simulink model "UNM_TrafficSignalFollower"  (R2025b)
settings: Solver=FixedStepAuto  StartTime=0  StopTime=1000  FixedStep=Ts  RelTol=1e-3
PostLoadFcn:
  | UNM_Setup()
InitFcn:
  | rrHDMap = rrSim.get("Map");
values from neighbouring files (symbols this model uses):
  Ts = 0.1    [SurrogateTrafficEnv.m]    (also in SurrogateTrafficEnvACC.m; UNMTrafficSignalFollower_Block.m; UNM_AccelToSpeed.m; UNM_TrafficSignalVisualization.m = 0.05)
undefined symbols (not defined in the file or in its folder): ActorRuntime, Defined, Ego, Lane, m, n, User
libraries: roadrunnerscenario x11, rllib x1
CloseFcn:
  | clear egoActorID signalID Ts
settings Model: Creator=user  LastModifiedBy=user
settings DataIOCC: InspectSignalLogs=on
settings DebuggingCC: AlgebraicLoopMsg=none

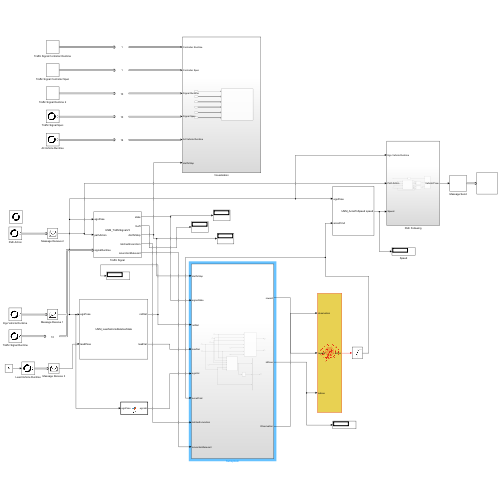
[thumbnail: Simulink's stored preview of the top-level diagram]
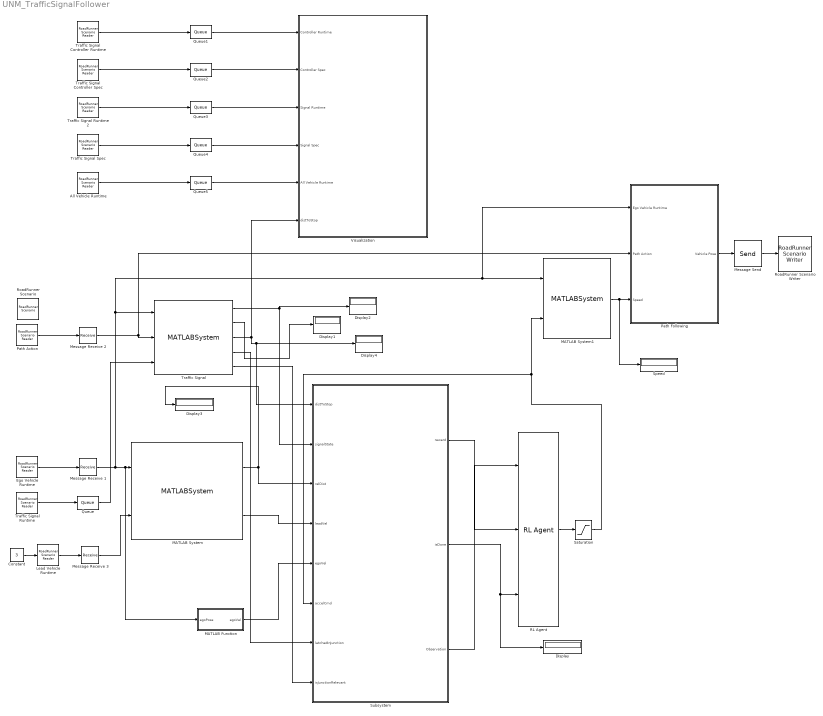
== system UNM_TrafficSignalFollower ==
  All Vehicle Runtime : roadrunnerscenario/RoadRunner Scenario Reader  TopicCategory=Actor  ActorCategory=Vehicle  ActionType=Path Following  EventType=User-Defined  TopicType=Actor Specifications  VehicleType=Vehicle Pose  TrafficSignalType=Traffic Signal Runtime  TrafficSignalControllerType=Traffic Signal Controller Specifications  UserDefinedAction=Action1  UserDefinedEvent=Event1  Filter=None  AdditionalRelationship=None  SensorTopic=Target Poses  LaneBoundaryOutputTopic=Ego-Lane  SensorID=1  SampleTime=Ts
  Constant : Constant  Value=3  OutDataTypeStr=uint64
  Display{,1..4} (5 alike) : Display
  Ego Vehicle Runtime : roadrunnerscenario/RoadRunner Scenario Reader  TopicCategory=Actor  ActorCategory=Vehicle  ActionType=Path Following  EventType=User-Defined  TopicType=Actor Specifications  VehicleType=Vehicle Pose  TrafficSignalType=Traffic Signal Specifications  TrafficSignalControllerType=Traffic Signal Controller Specifications  UserDefinedAction=Action1  UserDefinedEvent=Event1  Filter=Self  AdditionalRelationship=None  SensorTopic=Target Poses  LaneBoundaryOutputTopic=Ego-Lane  SensorID=1  SampleTime=Ts
  Lead Vehicle Runtime : roadrunnerscenario/RoadRunner Scenario Reader  TopicCategory=Actor  ActorCategory=Vehicle  ActionType=Path Following  EventType=User-Defined  TopicType=Actor Specifications  VehicleType=Vehicle Pose  TrafficSignalType=Traffic Signal Specifications  TrafficSignalControllerType=Traffic Signal Controller Specifications  UserDefinedAction=Action1  UserDefinedEvent=Event1  Filter=Actor ID (provided by input)  AdditionalRelationship=None  SensorTopic=Target Poses  LaneBoundaryOutputTopic=Ego-Lane  SensorID=1  SampleTime=Ts
  MATLAB Function : MATLAB Function  TreatAsAtomicUnit=on
  MATLAB System : MATLABSystem  System=UNM_LeadVehicleRelativeState
      mask Type: UNM_LeadVehicleRelativeState
  MATLAB System1 : MATLABSystem  System=UNM_AccelToSpeed  Ts=0.1  MaxSpeed=15
      mask Type: UNM_AccelToSpeed
  "Message Receive 1 " : Receive  InputPortMessageModes=m  UseInternalQueue=off  QueueOverwriting=on  QueueLength=1  QueueType=LIFO
  Message Receive 2 : Receive  InputPortMessageModes=m
  Message Receive 3 : Receive  InputPortMessageModes=m  UseInternalQueue=off  QueueOverwriting=on  QueueLength=1  QueueType=LIFO
  Message Send : Send  OutputPortMessageModes=m
  Path Action : roadrunnerscenario/RoadRunner Scenario Reader  TopicCategory=Action  ActorCategory=All Types  ActionType=Path Following  EventType=User-Defined  TopicType=Actor Specifications  VehicleType=Vehicle Specifications  TrafficSignalType=Traffic Signal Specifications  TrafficSignalControllerType=Traffic Signal Controller Specifications  UserDefinedAction=Action1  UserDefinedEvent=Event1  Filter=Self  AdditionalRelationship=None  SensorTopic=Target Poses  LaneBoundaryOutputTopic=Ego-Lane  SensorID=1  SampleTime=Ts
  Path Following : Subsystem
  Queue : Queue  InputPortMessageModes=m  OutputPortMessageModes=m  OverwriteOldest=on  Capacity=10
  Queue1 : Queue  InputPortMessageModes=m  OutputPortMessageModes=m  OverwriteOldest=on  Capacity=1
  Queue2 : Queue  InputPortMessageModes=m  OutputPortMessageModes=m  OverwriteOldest=on  Capacity=1
  Queue3 : Queue  InputPortMessageModes=m  OutputPortMessageModes=m  OverwriteOldest=on  Capacity=10
  Queue4 : Queue  InputPortMessageModes=m  OutputPortMessageModes=m  OverwriteOldest=on  Capacity=10
  Queue5 : Queue  InputPortMessageModes=m  OutputPortMessageModes=m  OverwriteOldest=on  Capacity=16
  RL Agent : rllib/RL Agent  Agent=agent  ExternalActionAsInput=off  ProvideLastAction=off  ProvideCumRwd=off  TreatAsDirectFeedthrough=on  UseStrictObservationDataTypes=off
  RoadRunner Scenario : roadrunnerscenario/RoadRunner Scenario  UserDefinedActions={}  UserDefinedEvents={}  PathPoints=500
  RoadRunner Scenario Writer : roadrunnerscenario/RoadRunner Scenario Writer  TopicCategory=Actor  ActorCategory=Vehicle  EventType=Action Complete  UserDefinedEvent=Event1  VehicleType=Vehicle Pose  TopicType=Actor Pose
  Saturation : Saturate  UpperLimit=2  LowerLimit=-3
  Speed : Display
  Subsystem : Subsystem
  Traffic Signal : MATLABSystem  InputPortMessageModes=n,n,m  System=UNM_TrafficSignalV3  SignalID=signalID  EgoID=egoActorID  RRHDMap=rrHDMap  MaxStopDistance=100  MaxPhaseDuration=60
      mask Type: UNM_TrafficSignalV3
  Traffic Signal Controller Runtime : roadrunnerscenario/RoadRunner Scenario Reader  TopicCategory=Actor  ActorCategory=Traffic Signal Controller  ActionType=Path Following  EventType=User-Defined  TopicType=Actor Specifications  VehicleType=Vehicle Pose  TrafficSignalType=Traffic Signal Runtime  TrafficSignalControllerType=Traffic Signal Controller Runtime  UserDefinedAction=Action1  UserDefinedEvent=Event1  Filter=None  AdditionalRelationship=None  SensorTopic=Target Poses  LaneBoundaryOutputTopic=Ego-Lane  SensorID=1  SampleTime=Ts
  Traffic Signal Controller Spec : roadrunnerscenario/RoadRunner Scenario Reader  TopicCategory=Actor  ActorCategory=Traffic Signal Controller  ActionType=Path Following  EventType=User-Defined  TopicType=Actor Specifications  VehicleType=Vehicle Pose  TrafficSignalType=Traffic Signal Runtime  TrafficSignalControllerType=Traffic Signal Controller Specifications  UserDefinedAction=Action1  UserDefinedEvent=Event1  Filter=None  AdditionalRelationship=None  SensorTopic=Target Poses  LaneBoundaryOutputTopic=Ego-Lane  SensorID=1  SampleTime=10
  Traffic Signal Runtime : roadrunnerscenario/RoadRunner Scenario Reader  TopicCategory=Actor  ActorCategory=Traffic Signal  ActionType=Path Following  EventType=User-Defined  TopicType=Actor Specifications  VehicleType=Vehicle Pose  TrafficSignalType=Traffic Signal Runtime  TrafficSignalControllerType=Traffic Signal Controller Specifications  UserDefinedAction=Action1  UserDefinedEvent=Event1  Filter=None  AdditionalRelationship=None  SensorTopic=Target Poses  LaneBoundaryOutputTopic=Ego-Lane  SensorID=1  SampleTime=Ts
  Traffic Signal Runtime 2 : roadrunnerscenario/RoadRunner Scenario Reader  TopicCategory=Actor  ActorCategory=Traffic Signal  ActionType=Path Following  EventType=User-Defined  TopicType=Actor Specifications  VehicleType=Vehicle Pose  TrafficSignalType=Traffic Signal Runtime  TrafficSignalControllerType=Traffic Signal Controller Specifications  UserDefinedAction=Action1  UserDefinedEvent=Event1  Filter=None  AdditionalRelationship=None  SensorTopic=Target Poses  LaneBoundaryOutputTopic=Ego-Lane  SensorID=1  SampleTime=Ts
  Traffic Signal Spec : roadrunnerscenario/RoadRunner Scenario Reader  TopicCategory=Actor  ActorCategory=Traffic Signal  ActionType=Path Following  EventType=User-Defined  TopicType=Actor Specifications  VehicleType=Vehicle Pose  TrafficSignalType=Traffic Signal Specifications  TrafficSignalControllerType=Traffic Signal Controller Specifications  UserDefinedAction=Action1  UserDefinedEvent=Event1  Filter=None  AdditionalRelationship=None  SensorTopic=Target Poses  LaneBoundaryOutputTopic=Ego-Lane  SensorID=1  SampleTime=10
  Visualization : Subsystem
  wires:
  Traffic Signal Spec/1 -> Queue4/1
  Message Receive 2/1 -> Path Following/2(Path Action), Traffic Signal/2
  Traffic Signal Runtime 2/1 -> Queue3/1
  Traffic Signal Runtime/1 -> Queue/1
  Message Send/1 -> RoadRunner Scenario Writer/1
  Path Action/1 -> Message Receive 2/1
  Ego Vehicle Runtime/1 -> "Message Receive 1 "/1
  Traffic Signal Controller Spec/1 -> Queue2/1
  "Message Receive 1 "/1 -> Path Following/1(Ego Vehicle Runtime), MATLAB System1/1, Traffic Signal/1, MATLAB Function/1(egoPose), MATLAB System/1
  Traffic Signal Controller Runtime/1 -> Queue1/1
  All Vehicle Runtime/1 -> Queue5/1
  Queue/1 -> Traffic Signal/3
  Queue1/1 -> Visualization/1(Controller Runtime)
  Queue2/1 -> Visualization/2(Controller Spec)
  Queue3/1 -> Visualization/3(Signal Runtime)
  RL Agent/1 -> Saturation/1
  Queue4/1 -> Visualization/4(Signal Spec)
  Traffic Signal/1 -> Subsystem/2(signalState), Display2/1
  Queue5/1 -> Visualization/5(All Vehicle Runtime)
  Saturation/1 -> MATLAB System1/2, Subsystem/6(accelCmd)
  Traffic Signal/2 -> Display1/1
  Traffic Signal/3 -> Subsystem/1(distToStop), Display4/1, Visualization/6(distToStop)
  MATLAB System/1 -> Display3/1, Subsystem/3(relDist)
  Subsystem/1(reward) -> RL Agent/2
  Subsystem/2(isDone) -> RL Agent/3, Display/1
  Subsystem/3(Observation) -> RL Agent/1
  MATLAB System1/1 -> Speed/1, Path Following/3(Speed)
  Path Following/1(Vehicle Pose) -> Message Send/1
  Constant/1 -> Lead Vehicle Runtime/1
  Lead Vehicle Runtime/1 -> Message Receive 3/1
  Message Receive 3/1 -> MATLAB System/2
  MATLAB System/2 -> Subsystem/4(leadVel)
  MATLAB Function/1(egoVel) -> Subsystem/5(egoVel)
  Traffic Signal/4 -> Subsystem/7(latchedInJunction)
  Traffic Signal/5 -> Subsystem/8(isJunctionRelevant)

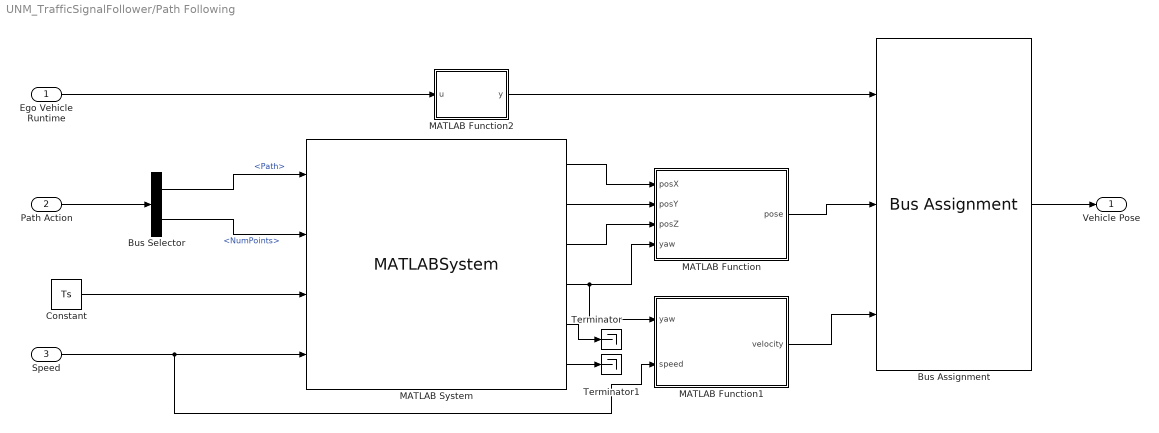
== system UNM_TrafficSignalFollower/Path Following ==
  Ego Vehicle Runtime : Inport
  Path Action : Inport  Port=2
  Speed : Inport  Port=3
  Bus Assignment : BusAssignment  AssignedSignals=ActorRuntime.Pose,ActorRuntime.Velocity
  Bus Selector : BusSelector  OutputSignals=PathTarget.Path,PathTarget.NumPoints
  Constant : Constant  Value=Ts
  MATLAB Function : MATLAB Function  TreatAsAtomicUnit=on
  MATLAB Function1 : MATLAB Function  TreatAsAtomicUnit=on
  MATLAB Function2 : MATLAB Function  TreatAsAtomicUnit=on
  MATLAB System : MATLABSystem  System=UNMPathEvaluator_Block  SimulateUsing=Code generation
      mask Type: UNMPathEvaluator_Block
  Terminator : Terminator
  Terminator1 : Terminator
  Vehicle Pose : Outport
  wires:
  Bus Assignment/1 -> Vehicle Pose/1
  Path Action/1 -> Bus Selector/1
  Constant/1 -> MATLAB System/3
  Speed/1 -> MATLAB Function1/2(speed), MATLAB System/4
  MATLAB Function1/1(velocity) -> Bus Assignment/3
  MATLAB System/1 -> MATLAB Function/1(posX)
  MATLAB Function/1(pose) -> Bus Assignment/2
  MATLAB System/2 -> MATLAB Function/2(posY)
  MATLAB System/3 -> MATLAB Function/3(posZ)
  MATLAB System/4 -> MATLAB Function/4(yaw), MATLAB Function1/1(yaw)
  MATLAB System/5 -> Terminator/1
  MATLAB System/6 -> Terminator1/1
  Bus Selector/1 -> MATLAB System/1  "<Path>"
  Bus Selector/2 -> MATLAB System/2  "<NumPoints>"
  Ego Vehicle Runtime/1 -> MATLAB Function2/1(u)
  MATLAB Function2/1(y) -> Bus Assignment/1

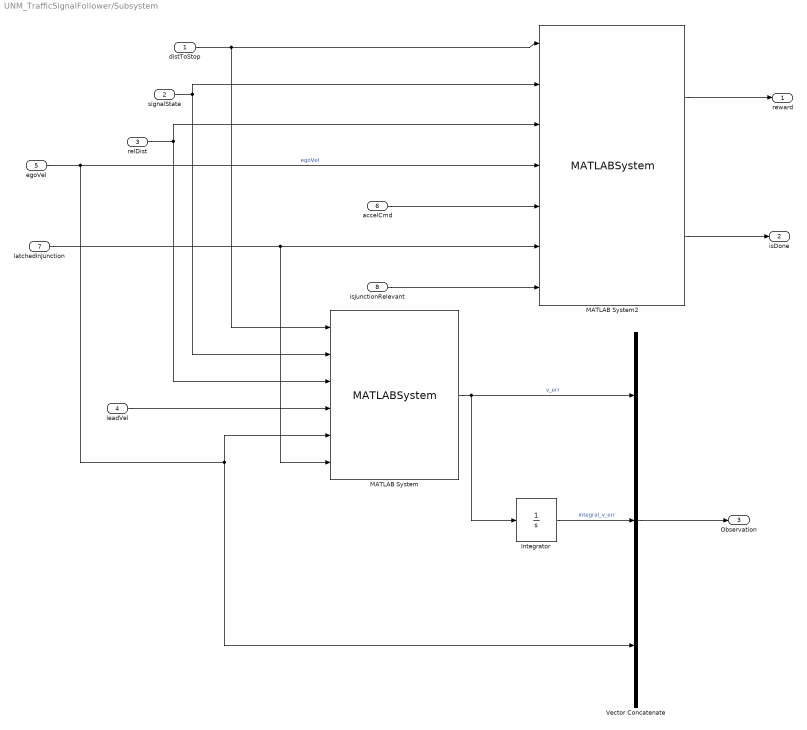
== system UNM_TrafficSignalFollower/Subsystem ==
  distToStop : Inport
  signalState : Inport  Port=2
  relDist : Inport  Port=3
  leadVel : Inport  Port=4
  egoVel : Inport  Port=5
  accelCmd : Inport  Port=6
  latchedInJunction : Inport  Port=7
  isJunctionRelevant : Inport  Port=8
  Integrator : Integrator
  MATLAB System : MATLABSystem  System=UNM_VRefCalculator  D_default=10  t_gap=1.4  v_set=30
      mask Type: UNM_VRefCalculator
  MATLAB System2 : MATLABSystem  System=UNM_RLRewardFcn  DesiredGap=10  CollisionGap=1.5  SignalViolationPenalty=100  CollisionPenalty=100  GapWeight=0.1  JerkWeight=0.05  SpeedWeight=0.01
      mask Type: UNM_RLRewardFcn
  Vector Concatenate : Concatenate  NumInputs=3
  reward : Outport
  isDone : Outport  Port=2
  Observation : Outport  Port=3
  wires:
  distToStop/1 -> MATLAB System/1, MATLAB System2/1
  signalState/1 -> MATLAB System/2, MATLAB System2/2
  relDist/1 -> MATLAB System/3, MATLAB System2/3
  leadVel/1 -> MATLAB System/4
  egoVel/1 -> Vector Concatenate/3, MATLAB System/5, MATLAB System2/4  "egoVel"
  MATLAB System2/2 -> isDone/1
  MATLAB System2/1 -> reward/1
  MATLAB System/1 -> Integrator/1, Vector Concatenate/1  "v_err"
  Vector Concatenate/1 -> Observation/1
  Integrator/1 -> Vector Concatenate/2  "integral_v_err"
  isJunctionRelevant/1 -> MATLAB System2/7
  accelCmd/1 -> MATLAB System2/5
  latchedInJunction/1 -> MATLAB System/6, MATLAB System2/6

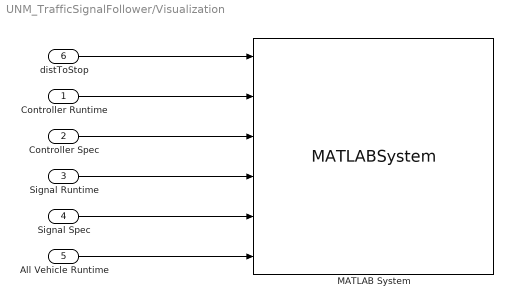
== system UNM_TrafficSignalFollower/Visualization ==
  Controller Runtime : Inport
  Controller Spec : Inport  Port=2
  Signal Runtime : Inport  Port=3
  Signal Spec : Inport  Port=4
  All Vehicle Runtime : Inport  Port=5
  distToStop : Inport  Port=6
  MATLAB System : MATLABSystem  InputPortMessageModes=n,m,m,m,m,m  System=UNM_TrafficSignalVisualization  RRHDMap=rrHDMap  VehicleSpec=vehicleSpec  EgoControllerID=controllerID  EgoSignalID=signalID  EgoID=egoActorID  Ts=Ts  DisableVisualization=off
      mask Type: UNM_TrafficSignalVisualization
  wires:
  distToStop/1 -> MATLAB System/1
  Controller Runtime/1 -> MATLAB System/2
  Controller Spec/1 -> MATLAB System/3
  Signal Runtime/1 -> MATLAB System/4
  Signal Spec/1 -> MATLAB System/5
  All Vehicle Runtime/1 -> MATLAB System/6

== matlab function UNM_TrafficSignalFollower/Path Following/MATLAB Function1 ==
  data: yaw input; velocity output; speed input
function velocity=getVehVel(yaw,speed)
% speed * direction unit vector = velocity vector 
    velocity = speed*[-sin(yaw) cos(yaw) 0];
end

== matlab function UNM_TrafficSignalFollower/Path Following/MATLAB Function ==
  data: posX input; pose output; posY input; posZ input; yaw input
function pose = packActorPose(posX, posY, posZ, yaw)
    % Pack the pose into 4x4 matrix.
    Position = [posX posY posZ];
    Rotation = [yaw 0 0];  % [yaw pitch roll] for vehicle pitch and roll are zero 
    % Get 3x3 rotation matrix
    rotm = eul2rotm(Rotation);            
    pose = [[rotm Position']; [0 0 0 1]];
end

== matlab function UNM_TrafficSignalFollower/Path Following/MATLAB Function2 ==
  data: u input Bus: BusVehicleRuntime; y output Bus: BusVehicleRuntime
function y = fcn(u)

y = u;

== matlab function UNM_TrafficSignalFollower/MATLAB Function ==
  data: egoPose input; egoVel output
function egoVel = fcn(egoPose)
    egoVel = norm(egoPose.ActorRuntime.Velocity);
end
